simulink model "TorqueSim"  (R2021a)
settings: Solver=VariableStepAuto  StartTime=0.0  StopTime=10.0  RelTol=1e-3
settings Model: Creator=johna  LastModifiedBy=johna

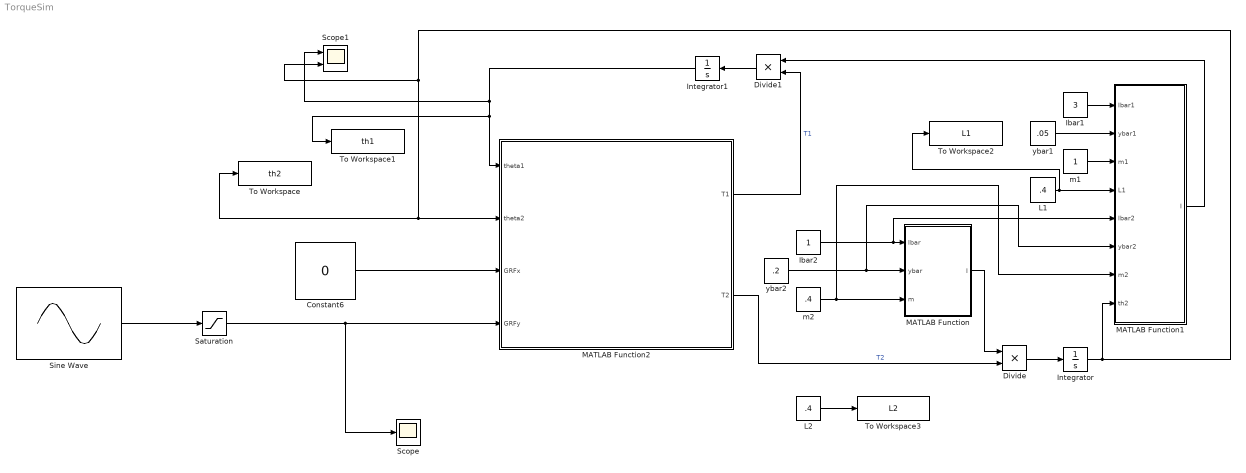
== system TorqueSim ==
  Constant6 : Constant  Value=0
  Divide : Product  Inputs=**
  Divide1 : Product  Inputs=**
  Ibar1 : Constant  Value=3
  Ibar2 : Constant
  Integrator : Integrator  InitialCondition=1.4
  Integrator1 : Integrator  InitialCondition=-.7
  L1 : Constant  Value=.4
  L2 : Constant  Value=.4
  MATLAB Function : MATLAB Function  TreatAsAtomicUnit=on
  MATLAB Function1 : MATLAB Function  TreatAsAtomicUnit=on
  MATLAB Function2 : MATLAB Function  TreatAsAtomicUnit=on
  Saturation : Saturate  UpperLimit=inf  LowerLimit=0
  Scope : Scope
  Scope1 : Scope  NumInputPorts=2
  Sine Wave : Sin  SampleTime=0
  To Workspace : ToWorkspace  VariableName=th2  SampleTime=-1
  To Workspace1 : ToWorkspace  VariableName=th1  SampleTime=-1
  To Workspace2 : ToWorkspace  VariableName=L1  SampleTime=-1
  To Workspace3 : ToWorkspace  VariableName=L2  SampleTime=-1
  m1 : Constant
  m2 : Constant  Value=.4
  ybar1 : Constant  Value=.05
  ybar2 : Constant  Value=.2
  wires:
  Constant6/1 -> MATLAB Function2/3(GRFx)
  Saturation/1 -> Scope/1, MATLAB Function2/4(GRFy)
  Sine Wave/1 -> Saturation/1
  Divide/1 -> Integrator/1
  Integrator/1 -> MATLAB Function1/8(th2), Scope1/2, To Workspace/1, MATLAB Function2/2(theta2)
  ybar1/1 -> MATLAB Function1/2(ybar1)
  Ibar1/1 -> MATLAB Function1/1(Ibar1)
  m1/1 -> MATLAB Function1/3(m1)
  L1/1 -> MATLAB Function1/4(L1), To Workspace2/1
  Ibar2/1 -> MATLAB Function1/5(Ibar2), MATLAB Function/1(Ibar)
  ybar2/1 -> MATLAB Function/2(ybar), MATLAB Function1/6(ybar2)
  m2/1 -> MATLAB Function1/7(m2), MATLAB Function/3(m)
  MATLAB Function2/2(T2) -> Divide/2  "T2"
  MATLAB Function/1(I) -> Divide/1
  Divide1/1 -> Integrator1/1
  MATLAB Function1/1(I) -> Divide1/1
  MATLAB Function2/1(T1) -> Divide1/2  "T1"
  Integrator1/1 -> Scope1/1, To Workspace1/1, MATLAB Function2/1(theta1)
  L2/1 -> To Workspace3/1

== matlab function TorqueSim/MATLAB Function1 ==
  data: Ibar1 input; I output; ybar1 input; m1 input; L1 input; Ibar2 input; ybar2 input; m2 input; th2 input
function I = fcn(Ibar1,ybar1,m1,L1,Ibar2, ybar2,m2,th2)
I = Ibar1 + ybar1^2 * m1 + Ibar2 + m2*sqrt((L1 + ybar2*cos(th2))^2 + (ybar2*sin(th2))^2);

== matlab function TorqueSim/MATLAB Function ==
  data: Ibar input; I output; ybar input; m input
function I = fcn(Ibar,ybar,m)
I = Ibar + ybar^2 * m

== matlab function TorqueSim/MATLAB Function2 ==
  data: theta1 input; T1 output; theta2 input; GRFx input; GRFy input; T2 output
function [T1, T2] = getTorque(theta1, theta2, GRFx, GRFy)
% t = 1:0.05:4;
% f = 0.5;
% y=sin(2*pi*f*t);% Generate Sine Wave  
% y(y<0) = 0;                       % Rectified Sine Wave
% plot(t,y);
if isempty(theta1)
    theta1 = 0;
end
if isempty(theta2)
    theta2 = 0;
end

F = [GRFx
     GRFy];

L1 = 2; 
L2 = 3; 
J = [(L1 * cos(theta1) + L2 * cos(theta1-theta2)) (L2 * cos(theta1-theta2))
         (-L1 * sin(theta1) - L2 * cos(theta1-theta2))  (-L2 * sin(theta1-theta2))];
     
   
T = ((J')^-1)\F;
T1 = T(1); 
T2 = T(2);
